simulink model "sim1"  (R2021b)
settings: Solver=VariableStepAuto  StartTime=0.0  StopTime=30.0  RelTol=1e-3
settings Model: Creator=dcheb  LastModifiedBy=dcheb

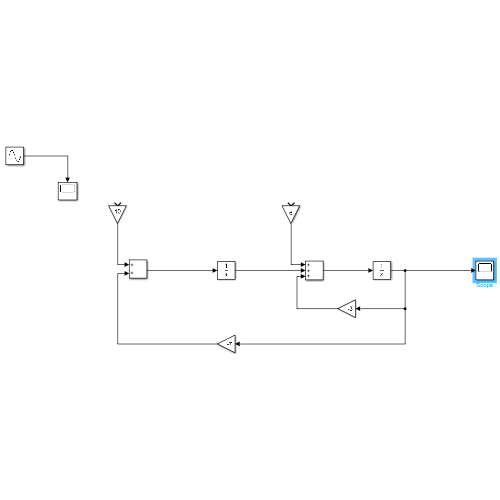
[thumbnail: Simulink's stored preview of the top-level diagram]
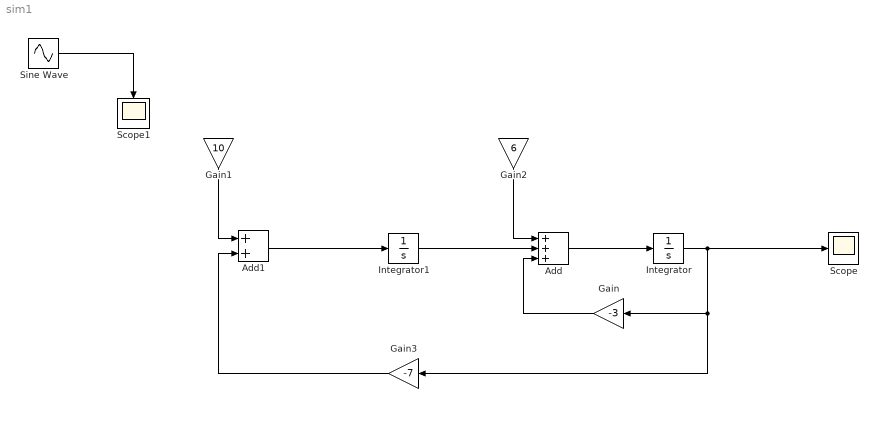
== system sim1 ==
  Add : Sum  Inputs=+++
  Add1 : Sum
  Gain : Gain  Gain=-3
  Gain1 : Gain  Gain=10
  Gain2 : Gain  Gain=6
  Gain3 : Gain  Gain=-7
  Integrator : Integrator  InitialCondition=1
  Integrator1 : Integrator  InitialCondition=3.4
  Scope : Scope
  Scope1 : Scope
  Sine Wave : Sin  Amplitude=2  SampleTime=0
  wires:
  Gain1/1 -> Add1/1
  Gain2/1 -> Add/1
  Add1/1 -> Integrator1/1
  Integrator1/1 -> Add/2
  Add/1 -> Integrator/1
  Integrator/1 -> Scope/1, Gain/1, Gain3/1
  Gain3/1 -> Add1/2
  Gain/1 -> Add/3
  Sine Wave/1 -> Scope1/1
